simulink model "HVDCMMCInterconnection_O"  (R2023b)
settings: Solver=FixedStepDiscrete  StartTime=0.0  StopTime=10  RelTol=1e-3  EnableMultiTasking=on
PreLoadFcn:
  | HVDCMMCInterconnectionParam
StartFcn:
  | tic
StopFcn:
  | toc
values from neighbouring files (symbols this model uses):
  C_PM = 1.758e-3    (= 0.001758)    [HVDCMMCInterconnectionParam.m]
  Cfilter = 1/(Larm*wc2)    (= 4.78421193241e-05)    [HVDCMMCInterconnectionParam.m]
  Cg = 50e-9    (= 5e-08)    [HVDCMMCInterconnectionParam.m]
  Fc = Fnom*3.37    (= 168.5)    [HVDCMMCInterconnectionParam.m]
  Fnom = 50    [HVDCMMCInterconnectionParam.m]
  Ki_Ireg = 6    [HVDCMMCInterconnectionParam.m]
  Ki_Preg = 1.0    (= 1)    [HVDCMMCInterconnectionParam.m]
  Ki_Qreg = 1.0    (= 1)    [HVDCMMCInterconnectionParam.m]
  Ki_VDCreg = 100    [HVDCMMCInterconnectionParam.m]
  Kp_Ireg = 0.6    [HVDCMMCInterconnectionParam.m]
  Kp_Preg = 0.5/3    (= 0.166666666667)    [HVDCMMCInterconnectionParam.m]
  Kp_Qreg = 0.5/3    (= 0.166666666667)    [HVDCMMCInterconnectionParam.m]
  Kp_VDCreg = 4    [HVDCMMCInterconnectionParam.m]
  L_cable = 15e-3    (= 0.015)    [HVDCMMCInterconnectionParam.m]
  Larm = Larm_pu*(Zbase/(2*pi*Fnom))    (= 0.0529455974536)    [HVDCMMCInterconnectionParam.m]
  Lff = Larm_pu/2    (= 0.075)    [HVDCMMCInterconnectionParam.m]
  Limits_Ireg = [ 2.0  -2.0]    [HVDCMMCInterconnectionParam.m]
  Limits_Preg = [ 1.2, 0.8 ]    [HVDCMMCInterconnectionParam.m]
  Limits_Qreg = [ 0.25, -0.25 ]    [HVDCMMCInterconnectionParam.m]
  Limits_VDCreg = [ 2.0  -2.0]    [HVDCMMCInterconnectionParam.m]
  Lxfo = 0.12    [HVDCMMCInterconnectionParam.m]
  Nb_PM = 36    [HVDCMMCInterconnectionParam.m]
  Pnom = 1000e6    (= 1000000000)    [HVDCMMCInterconnectionParam.m]
  R_cable = 0.5    [HVDCMMCInterconnectionParam.m]
  R_startup = 400    [HVDCMMCInterconnectionParam.m]
  Rarm = Rarm_pu*Zbase    (= 0.1663335)    [HVDCMMCInterconnectionParam.m]
  Rff = Rarm_pu/2    (= 0.00075)    [HVDCMMCInterconnectionParam.m]
  Rfilter = 1/(Cfilter*w)*30    (= 1996.002)    [HVDCMMCInterconnectionParam.m]
  Rg = 100    [HVDCMMCInterconnectionParam.m]
  Rxfo = 0.003    [HVDCMMCInterconnectionParam.m]
  Slope_Pref = 0.5    [HVDCMMCInterconnectionParam.m]
  Slope_Qref = 0.5    [HVDCMMCInterconnectionParam.m]
  Slope_Vdc_ref = Vnom_dc/5    (= 128000)    [HVDCMMCInterconnectionParam.m]
  Tbrk1_On = 0.1    [HVDCMMCInterconnectionParam.m]
  Tbrk2_On = 1.0    (= 1)    [HVDCMMCInterconnectionParam.m]
  Tdeblock = 1.5    [HVDCMMCInterconnectionParam.m]
  Tfault = 9999    [HVDCMMCInterconnectionParam.m]
  Ton_Converter2 = 4    [HVDCMMCInterconnectionParam.m]
  Ton_PQreg = 4    [HVDCMMCInterconnectionParam.m]
  Ton_VDCreg = 1.5    [HVDCMMCInterconnectionParam.m]
  Ts = Ts_Control    (= 4e-05)    [HVDCMMCInterconnectionParam.m]
  Ts_Control = 40e-6    (= 4e-05)    [HVDCMMCInterconnectionParam.m]
  Ts_Power = 20e-6    (= 2e-05)    [HVDCMMCInterconnectionParam.m]
  Vnom_dc = 640e3    (= 640000)    [HVDCMMCInterconnectionParam.m]
  Vnom_prim = 400e3    (= 400000)    [HVDCMMCInterconnectionParam.m]
  Vnom_sec = 333e3    (= 333000)    [HVDCMMCInterconnectionParam.m]
undefined symbols (not defined in the file or in its folder): DiscIntNeverNeededParam, Pcc
libraries: spsSeriesRLCBranchLib x24, spsCurrentMeasurementLib x11, spsVoltageMeasurementLib x8, simulink x7, spsHalfBridgeMMCLib x6, powerlib_extras x3, spsIdealSwitchLib x3, spsBreakerLib x3, spsParallelRLCBranchLib x3, spsThreePhaseBreakerLib x2, spsMeanLib x2, spsSecondOrderFilterLib x2
(part 1 of 2)
settings Model: SimulationMode=accelerator  Creator=The MathWorks, Inc.  LastModifiedBy=The MathWorks, Inc.
settings SolverCC: AlgebraicLoopSolver=TrustRegion
settings DataIOCC: SaveFormat=StructureWithTime  SaveOutput=off  SignalLogging=off  DSMLogging=off  SaveTime=off  ReturnWorkspaceOutputs=off
settings OptimizationCC: ReuseModelBlockBuffer=off  ExpressionDepthLimit=2147483647  LifeSpan=inf
settings DebuggingCC: UnderspecifiedInitializationDetection=Classic  MergeDetectMultiDrivingBlocksExec=none  SolverPrmCheckMsg=warning  FcnCallInpInsideContextMsg=warning  UnconnectedInputMsg=warning  UnconnectedOutputMsg=warning  UnconnectedLineMsg=warning  AllowSymbolicDim=off  StateNameClashWarn=warning  SFUnexpectedBacktrackingDiag=warning  SFNoUnconditionalDefaultTransitionDiag=warning  SFExecutionAtInitializationDiag=none  ArithmeticOperatorsInVariantConditions=warning
settings HardwareCC: ProdBitPerPointer=32  ProdBitPerSizeT=32  ProdBitPerPtrDiffT=32  ProdLargestAtomicFloat=None  ProdIntDivRoundTo=Undefined  ProdEndianess=Unspecified  ProdWordSize=32  ProdHWDeviceType=32-bit Generic
settings ModelReferenceCC: EnableRefExpFcnMdlSchedulingChecks=on  PropagateSignalLabelsOutOfModel=off
settings SFSimCC: SimUseLocalCustomCode=off  CustomCodeUndefinedFunction=UseInterfaceOnly
settings RTWCC: RTWUseLocalCustomCode=off
settings CodeAppCC: StateflowObjectComments=on
settings GRTTargetCC: TargetLangStandard=C89/C90 (ANSI)  CombineOutputUpdateFcns=off  GRTInterface=on
settings ConfigComp: CovMetricSettings=dw  CovSaveCumulativeToWorkspaceVar=on  CovSaveSingleToWorkspaceVar=on  CovExternalEMLEnable=off
settings SimscapeCC: SimscapeNormalizeSystem=off

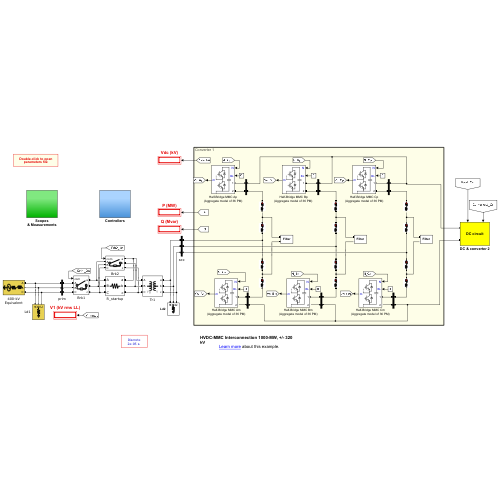
[thumbnail: Simulink's stored preview of the top-level diagram]
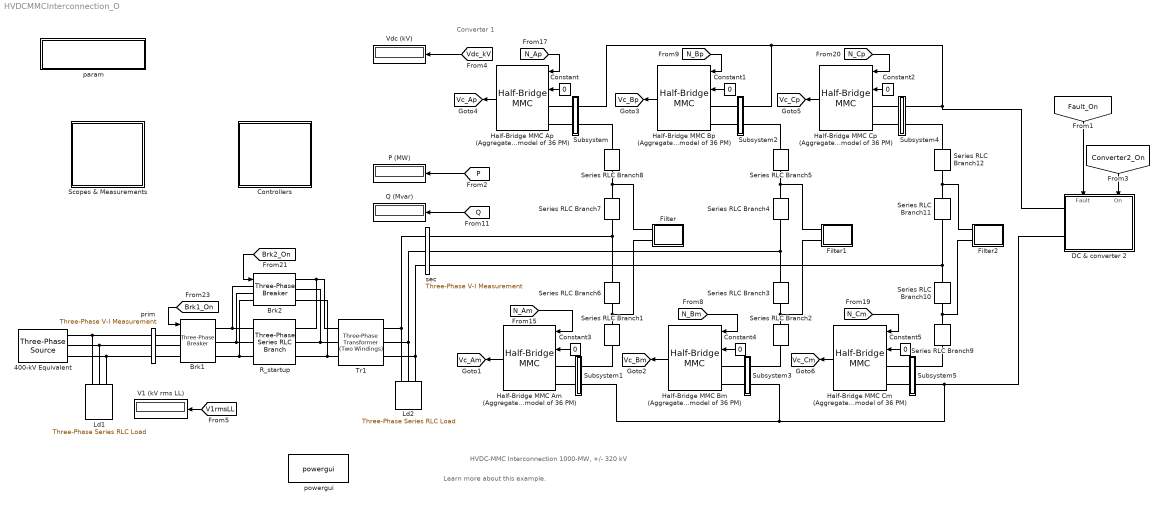
== system HVDCMMCInterconnection_O ==
  note: Converter 1
  note: HVDC-MMC Interconnection 1000-MW, +/- 320 kV
  note: Learn more about this example.
  400-kV Equivalent : spsThreePhaseSourceLib/Three-Phase Source  InternalConnection=Yg  VoltagePhases=off  Voltage=Vnom_prim*0.99  PhaseAngle=0  Voltage_phases=[25e3 25e3 25e3]/sqrt(3)  PhaseAngles_phases=[0 -120 +120]  Frequency=Fnom  NonIdealSource=on  SpecifyImpedance=on  Resistance=0.8929  Inductance=16.58e-3  ShortCircuitLevel=Psc  BaseVoltage=Vnom_prim  XRratio=7  BusType=swing  Pref=0  Qref=0  Prefabc=[10e3, 10e3, 10e3]  Qrefabc=[0, 0, 0]  Qmin=-inf  Qmax=inf
  Brk1 : spsThreePhaseBreakerLib/Three-Phase Breaker  InitialState=open  SwitchA=on  SwitchB=on  SwitchC=on  SwitchTimes=0.1  External=on  BreakerResistance=0.001  SnubberResistance=1e6  SnubberCapacitance=inf  Measurements=None
  Brk2 : spsThreePhaseBreakerLib/Three-Phase Breaker  InitialState=open  SwitchA=on  SwitchB=on  SwitchC=on  SwitchTimes=[30/60]*10000  External=on  BreakerResistance=0.01  SnubberResistance=1e6  SnubberCapacitance=inf  Measurements=None
  Constant{,1..5} (6 alike) : Constant  Value=0
  Controllers : Subsystem
  DC & converter 2 : Subsystem
      settings: PortSchema="{\"entries\":[{\"content\":{\"sides\":[{\"content\":{\"connectorIds\":[\"LConn1\",\"LConn2\"]},\"type\":\"ConnectorPlacement.EquallySpacedRectSide\",\"uuid\":\"7a2c87ad-91de-4512-ad2a-35713ffc2c67\"},{\"content\":{\"connectorIds\":[],\"side\":\"RIGHT\"},\"type\":\"ConnectorPlacement.EquallySpacedRectSide\",\"uuid\":\"a4d51b8d-9b80-4f56-8990-d227af10d4d9\"},{\"content\":{\"connectorIds\":[\"In1\",\"In2\"],\"side\":\"TOP\"},\"type\":\"ConnectorPlacement.EquallySpacedRectSide\",\"uuid\":\"21e823e1-439d-404c-83ef-6279f9df48a0\"}]},\"type\":\"ConnectorPlacement.EquallySpacedConnector\",\"uuid\":\"7be36849-7bc6-4892-aa95-a5e675f45e41\"}],\"packageUris\":[\"http://schema.mathworks.com/mf0/Connector/R2020b\"],\"version\":\"1.0\"}"
      mask Display: disp('DC circuit')
  Filter : Subsystem
      mask Display: disp('Filter')
  Filter1 : Subsystem
      mask Display: disp('Filter')
  Filter2 : Subsystem
      mask Display: disp('Filter')
  Half-Bridge MMC Am (Aggregate model of 36 PM) : spsHalfBridgeMMCLib/Half-Bridge MMC  ModelType=Aggregate model  n=36  C=C_PM  Vc_Initial=Vc0_PM  Ron=1e-3  Rs=1e6  Cs=inf  Ron_Diode=1e-3  Rs_Diode=1e6  Cs_Diode=inf  Vf_Diode=1e-3  Rs_CurrentSource=inf  Ts=Ts_Power
  Half-Bridge MMC Ap (Aggregate model of 36 PM) : spsHalfBridgeMMCLib/Half-Bridge MMC  ModelType=Aggregate model  n=36  C=C_PM  Vc_Initial=Vc0_PM  Ron=1e-3  Rs=1e6  Cs=inf  Ron_Diode=1e-3  Rs_Diode=1e6  Cs_Diode=inf  Vf_Diode=1e-3  Rs_CurrentSource=inf  Ts=Ts_Power
  Half-Bridge MMC Bm (Aggregate model of 36 PM) : spsHalfBridgeMMCLib/Half-Bridge MMC  ModelType=Aggregate model  n=36  C=C_PM  Vc_Initial=Vc0_PM  Ron=1e-3  Rs=1e6  Cs=inf  Ron_Diode=1e-3  Rs_Diode=1e6  Cs_Diode=inf  Vf_Diode=1e-3  Rs_CurrentSource=inf  Ts=Ts_Power
  "Half-Bridge MMC Bp (Aggregate model of 36 PM) " : spsHalfBridgeMMCLib/Half-Bridge MMC  ModelType=Aggregate model  n=36  C=C_PM  Vc_Initial=Vc0_PM  Ron=1e-3  Rs=1e6  Cs=inf  Ron_Diode=1e-3  Rs_Diode=1e6  Cs_Diode=inf  Vf_Diode=1e-3  Rs_CurrentSource=inf  Ts=Ts_Power
  Half-Bridge MMC Cm (Aggregate model of 36 PM) : spsHalfBridgeMMCLib/Half-Bridge MMC  ModelType=Aggregate model  n=36  C=C_PM  Vc_Initial=Vc0_PM  Ron=1e-3  Rs=1e6  Cs=inf  Ron_Diode=1e-3  Rs_Diode=1e6  Cs_Diode=inf  Vf_Diode=1e-3  Rs_CurrentSource=inf  Ts=Ts_Power
  Half-Bridge MMC Cp (Aggregate model of 36 PM) : spsHalfBridgeMMCLib/Half-Bridge MMC  ModelType=Aggregate model  n=36  C=C_PM  Vc_Initial=Vc0_PM  Ron=1e-3  Rs=1e6  Cs=inf  Ron_Diode=1e-3  Rs_Diode=1e6  Cs_Diode=inf  Vf_Diode=1e-3  Rs_CurrentSource=inf  Ts=Ts_Power
  Ld1 : spsThreePhaseSeriesRLCLoadLib/Three-Phase Series RLC Load  LConnTagsString=A|B|C  Configuration=Y (grounded)  NominalVoltage=Vnom_prim  Vabc=[1e3 1e3 1e3]  Vabcp=[1e3 1e3 1e3]  NominalFrequency=Fnom  UnbalancedPower=off  ActivePower=P_Ld1  InductivePower=0  CapacitivePower=0  Pabc=[10e3 9e3 11e3]  QLabc=[100 90 110]  QCabc=[100 90 110]  Pabcp=[10e3 9e3 11e3]  QLabcp=[100 90 110]  QCabcp=[100 90 110]  Measurements=None  LoadType=constant Z
  Ld2 : spsThreePhaseSeriesRLCLoadLib/Three-Phase Series RLC Load  LConnTagsString=A|B|C  Configuration=Y (grounded)  NominalVoltage=Vnom_sec  Vabc=[1e3 1e3 1e3]  Vabcp=[1e3 1e3 1e3]  NominalFrequency=Fnom  UnbalancedPower=off  ActivePower=500e3  InductivePower=0  CapacitivePower=0  Pabc=[10e3 9e3 11e3]  QLabc=[100 90 110]  QCabc=[100 90 110]  Pabcp=[10e3 9e3 11e3]  QLabcp=[100 90 110]  QCabcp=[100 90 110]  Measurements=None  LoadType=constant Z
  P (MW) : Display
      settings: Format=bank  Decimation=5000
  Q (Mvar) : Display
      settings: Format=bank  Decimation=5000
  R_startup : spsThreePhaseSeriesRLCBranchLib/Three-Phase Series RLC Branch  LConnTagsString=A|B|C  RConnTagsString=A|B|C  BranchType=R  Resistance=R_startup  Inductance=Vnom_prim^2 / Pcc / (2*pi*Fnom)  Capacitance=1e-6  Measurements=None
  Scopes & Measurements : Subsystem
  Series RLC Branch{1..12} (12 alike) : spsSeriesRLCBranchLib/Series RLC Branch  LConnTagsString=__new0  RConnTagsString=__new0  BranchType=RL  Resistance=Rarm/2  Inductance=Larm/2  SetiL0=off  InitialCurrent=0  Capacitance=1e-6  Setx0=off  InitialVoltage=0  Measurements=None
  Subsystem : Subsystem
  Subsystem1 : Subsystem
  Subsystem2 : Subsystem
  Subsystem3 : Subsystem
  Subsystem4 : Subsystem
  Subsystem5 : Subsystem
  Tr1 : spsThreePhaseTransformerTwoWindingsLib/Three-Phase Transformer (Two Windings)  Winding1Connection=Yg  Winding2Connection=Y  CoreType=Three single-phase transformers  SetSaturation=off  Hysteresis=off  DataFile='hysteresis'  SetInitialFlux=off  Measurements=None  UNITS=pu  NominalPower=[ Pnom , Fnom ]  Winding1="[ Vnom_prim , Rxfo/2,  Lxfo/2 ]"  Winding2="[ Vnom_sec , Rxfo/2,  Lxfo/2 ]"  Rm=1000  Lm=1000  L0=0.5  Saturation=[ 0,0 ; 0.0024,1.2 ; 1.0,1.52 ]  InitialFluxes=[ 0.8 , -0.8 , 0.7 ]  BreakLoop=off  DiscreteSolver=Trapezoidal iterative  DataType=off  TransfoNumber=1
  V1 (kV rms LL) : Display
      settings: Format=bank  Decimation=5000
  Vdc (kV) : Display
      settings: Format=bank  Decimation=5000
  param : Subsystem
      settings: OpenFcn=open('HVDCMMCInterconnectionParam')
      mask Display: disp('Double-click to open\nparameters file')
  powergui : spspowerguiLib/powergui  Priority=1  SimulationMode=Discrete  SampleTime=Ts_Power  frequency=60  Iterations=50  frequencyindice=0  Pbase=100e6  ErrMax=1e-4  UnitsV=kV  UnitsW=MW  buscounter=0  FunctionMessages=off  echomessages=off  EnableUseOfTLC=off  CurrentSourceSwitches=off  DisableSnubberDevices=off  DisableRonSwitches=off  DisableVfSwitches=off  DisplayEquations=off  AutomaticDiscreteSolvers=off  SolverType=Tustin/Backward Euler (TBE)  Interpol=off  ExternalGateDelay=off  methode=off  Ts=10  x0status=blocks  SPID=off  SwTol=0  HookPort=off  NonlinearTolerance=1e-4  nMaxIteration=100  ContinueOnMaxIteration=off  RestoreLinks=warning  ResistiveCurrentMeasurement=off  Frange=[0:2:500]  Ylog=off  Xlog=on  ShowGrid=off  save=off  variable=ZData  structure=VIprim  ZoomFFT=on  StartTime=0.15  cycles=2  DisplayStyle=1  fundamental=50  FreqAxis=on  MaxFrequency=1000  frequencyindicesteady=1  RmsSteady=1  display=off
  prim : spsThreePhaseVIMeasurementLib/Three-Phase V-I Measurement  VoltageMeasurement=phase-to-ground  SetLabelV=on  LabelV=Vprim  Vpu=off  VpuLL=off  CurrentMeasurement=yes  SetLabelI=on  LabelI=Iprim  Ipu=off  Pbase=100e6  Vbase=500e3  OutputType=Complex  PhasorSimulation=off  PSBequivalent=0
  sec : spsThreePhaseVIMeasurementLib/Three-Phase V-I Measurement  VoltageMeasurement=phase-to-ground  SetLabelV=on  LabelV=Vsec  Vpu=off  VpuLL=off  CurrentMeasurement=yes  SetLabelI=on  LabelI=Isec  Ipu=off  Pbase=100e6  Vbase=500e3  OutputType=Complex  PhasorSimulation=off  PSBequivalent=0
  tag scope: Vc_Am=global, Vc_Ap=global, Vc_Bm=global, Vc_Bp=global, Vc_Cm=global, Vc_Cp=global
  wires:
  [P] -> P (MW)/1
  [N_Cp] -> Half-Bridge MMC Cp (Aggregate model of 36 PM)/1
  Half-Bridge MMC Cp (Aggregate model of 36 PM)/1 -> [Vc_Cp]
  Half-Bridge MMC Am (Aggregate model of 36 PM)/1 -> [Vc_Am]
  Half-Bridge MMC Bm (Aggregate model of 36 PM)/1 -> [Vc_Bm]
  Half-Bridge MMC Cm (Aggregate model of 36 PM)/1 -> [Vc_Cm]
  [N_Bm] -> Half-Bridge MMC Bm (Aggregate model of 36 PM)/1
  [Brk2_On] -> Brk2/1
  [Brk1_On] -> Brk1/1
  [Vdc_kV] -> Vdc (kV)/1
  [V1rmsLL] -> V1 (kV rms LL)/1
  [Q] -> Q (Mvar)/1
  Half-Bridge MMC Ap (Aggregate model of 36 PM)/1 -> [Vc_Ap]
  [Converter2_On] -> DC & converter 2/2(On)
  [Fault_On] -> DC & converter 2/1(Fault)
  [N_Ap] -> Half-Bridge MMC Ap (Aggregate model of 36 PM)/1
  [N_Am] -> Half-Bridge MMC Am (Aggregate model of 36 PM)/1
  "Half-Bridge MMC Bp (Aggregate model of 36 PM) "/1 -> [Vc_Bp]
  [N_Bp] -> "Half-Bridge MMC Bp (Aggregate model of 36 PM) "/1
  [N_Cm] -> Half-Bridge MMC Cm (Aggregate model of 36 PM)/1
  Constant/1 -> Half-Bridge MMC Ap (Aggregate model of 36 PM)/2
  Constant1/1 -> "Half-Bridge MMC Bp (Aggregate model of 36 PM) "/2
  Constant2/1 -> Half-Bridge MMC Cp (Aggregate model of 36 PM)/2
  Constant3/1 -> Half-Bridge MMC Am (Aggregate model of 36 PM)/2
  Constant4/1 -> Half-Bridge MMC Bm (Aggregate model of 36 PM)/2
  Constant5/1 -> Half-Bridge MMC Cm (Aggregate model of 36 PM)/2
  connections:
  400-kV Equivalent/RConn1 -- Ld1/LConn1 -- prim/RConn1
  400-kV Equivalent/RConn2 -- Ld1/LConn2 -- prim/RConn2
  400-kV Equivalent/RConn3 -- Ld1/LConn3 -- prim/RConn3
  Series RLC Branch7/RConn1 -- Series RLC Branch6/LConn1 -- sec/LConn1
  Series RLC Branch1/LConn1 -- Filter/LConn2 -- Series RLC Branch6/RConn1
  Series RLC Branch7/LConn1 -- Filter/LConn1 -- Series RLC Branch8/RConn1
  Half-Bridge MMC Ap (Aggregate model of 36 PM)/LConn1 -- Subsystem/LConn1
  Subsystem/LConn2 -- Half-Bridge MMC Ap (Aggregate model of 36 PM)/LConn2
  Subsystem/RConn2 -- Series RLC Branch8/LConn1
  Half-Bridge MMC Am (Aggregate model of 36 PM)/LConn2 -- Subsystem1/LConn2
  Half-Bridge MMC Am (Aggregate model of 36 PM)/LConn1 -- Subsystem1/LConn1
  Series RLC Branch1/RConn1 -- Subsystem1/RConn1
  Series RLC Branch4/RConn1 -- Series RLC Branch3/LConn1 -- sec/LConn2
  Filter1/LConn2 -- Series RLC Branch2/LConn1 -- Series RLC Branch3/RConn1
  Series RLC Branch4/LConn1 -- Filter1/LConn1 -- Series RLC Branch5/RConn1
  "Half-Bridge MMC Bp (Aggregate model of 36 PM) "/LConn2 -- Subsystem2/LConn2
  "Half-Bridge MMC Bp (Aggregate model of 36 PM) "/LConn1 -- Subsystem2/LConn1
  Subsystem2/RConn2 -- Series RLC Branch5/LConn1
  Series RLC Branch2/RConn1 -- Subsystem3/RConn1
  Half-Bridge MMC Bm (Aggregate model of 36 PM)/LConn1 -- Subsystem3/LConn1
  Half-Bridge MMC Bm (Aggregate model of 36 PM)/LConn2 -- Subsystem3/LConn2
  Series RLC Branch11/RConn1 -- Series RLC Branch10/LConn1 -- sec/LConn3
  Series RLC Branch10/RConn1 -- Filter2/LConn2 -- Series RLC Branch9/LConn1
  Series RLC Branch12/RConn1 -- Series RLC Branch11/LConn1 -- Filter2/LConn1
  Half-Bridge MMC Cp (Aggregate model of 36 PM)/LConn1 -- Subsystem4/LConn1
  Half-Bridge MMC Cm (Aggregate model of 36 PM)/LConn1 -- Subsystem5/LConn1
  Half-Bridge MMC Cm (Aggregate model of 36 PM)/LConn2 -- Subsystem5/LConn2
  Subsystem4/RConn2 -- Series RLC Branch12/LConn1
  Half-Bridge MMC Cp (Aggregate model of 36 PM)/LConn2 -- Subsystem4/LConn2
  Series RLC Branch9/RConn1 -- Subsystem5/RConn1
  Subsystem/RConn1 -- Subsystem4/RConn1 -- DC & converter 2/LConn1 -- Subsystem2/RConn1
  Subsystem1/RConn2 -- Subsystem5/RConn2 -- DC & converter 2/LConn2 -- Subsystem3/RConn2
  sec/RConn1 -- Ld2/LConn1 -- Tr1/RConn1
  sec/RConn2 -- Ld2/LConn2 -- Tr1/RConn2
  sec/RConn3 -- Ld2/LConn3 -- Tr1/RConn3
  Brk2/LConn1 -- R_startup/LConn1 -- Brk1/RConn1
  Brk1/RConn2 -- Brk2/LConn2 -- R_startup/LConn2
  Brk1/RConn3 -- Brk2/LConn3 -- R_startup/LConn3
  R_startup/RConn1 -- Brk2/RConn1 -- Tr1/LConn1
  R_startup/RConn2 -- Brk2/RConn2 -- Tr1/LConn2
  R_startup/RConn3 -- Brk2/RConn3 -- Tr1/LConn3
  prim/LConn1 -- Brk1/LConn1
  prim/LConn2 -- Brk1/LConn2
  prim/LConn3 -- Brk1/LConn3

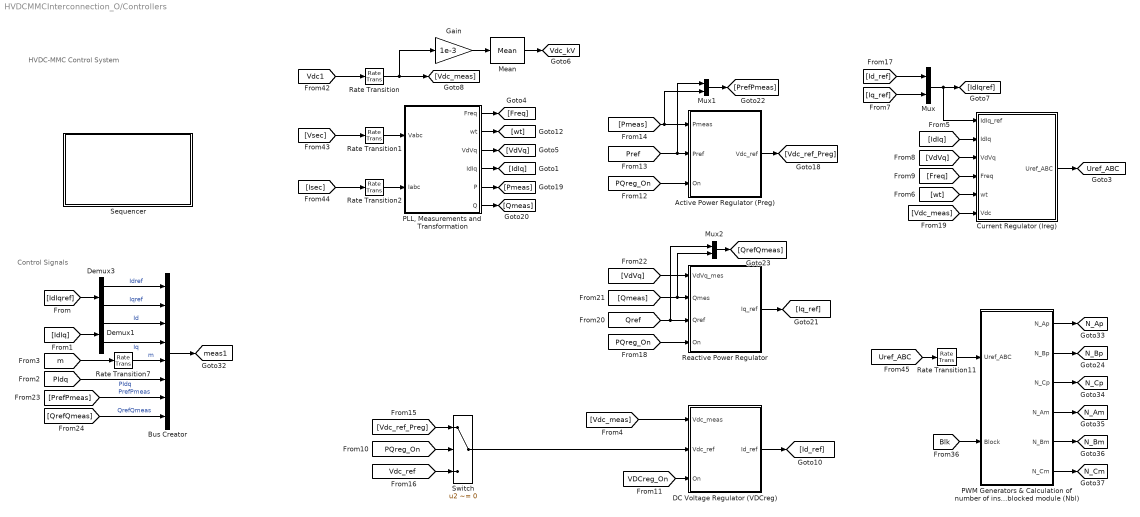
== system HVDCMMCInterconnection_O/Controllers ==
  note: HVDC-MMC Control System
  note: Control Signals
  Active Power Regulator (Preg) : Subsystem
  Bus Creator : BusCreator  Inputs=8
  Current Regulator (Ireg) : Subsystem
  DC Voltage Regulator (VDCreg) : Subsystem
  Demux1 : Demux  Outputs=2
  Demux3 : Demux  Outputs=2
  Gain : Gain  Gain=1e-3
  Mean : spsMeanLib/Mean  Freq=Fnom/3  Vinit=0  Ts=Ts_Control
  Mux : Mux  Inputs=2
  Mux1 : Mux  Inputs=2
  Mux2 : Mux  Inputs=2
  "PLL, Measurements and Transformation" : Subsystem
  PWM Generators & Calculation of number of inserted modules (Nin) and number of blocked module (Nbl) : Subsystem
  Rate Transition{,1..2,7} (4 alike) : RateTransition  OutPortSampleTime=Ts_Control
  Rate Transition11 : RateTransition  OutPortSampleTime=Ts_Power
  Reactive Power Regulator : Subsystem
  Sequencer : Subsystem
      mask Display: disp('Sequencer')
  Switch : Switch  Criteria=u2 ~= 0  SaturateOnIntegerOverflow=off  InputSameDT=off
  tag scope: N_Am=global, N_Ap=global, N_Bm=global, N_Bp=global, N_Cm=global, N_Cp=global, Uref_ABC=global, Vdc_kV=global, meas1=global
  wires:
  Rate Transition11/1 -> PWM Generators & Calculation of number of inserted modules (Nin) and number of blocked module (Nbl)/1(Uref_ABC)
  [Uref_ABC] -> Rate Transition11/1
  Mean/1 -> [Vdc_kV]
  [Vsec] -> Rate Transition1/1
  [Isec] -> Rate Transition2/1
  [Vdc_meas] -> Current Regulator (Ireg)/6(Vdc)
  [Vdc_meas] -> DC Voltage Regulator (VDCreg)/1(Vdc_meas)
  DC Voltage Regulator (VDCreg)/1(Id_ref) -> [Id_ref]
  Gain/1 -> Mean/1
  Current Regulator (Ireg)/1(Uref_ABC) -> [Uref_ABC]
  [wt] -> Current Regulator (Ireg)/5(wt)
  [Vdc1] -> Rate Transition/1
  "PLL, Measurements and Transformation"/2(wt) -> [wt]
  "PLL, Measurements and Transformation"/4(IdIq) -> [IdIq]
  [Freq] -> Current Regulator (Ireg)/4(Freq)
  [Id_ref] -> Mux/1
  "PLL, Measurements and Transformation"/3(VdVq) -> [VdVq]
  Mux/1 -> Current Regulator (Ireg)/1(IdIq_ref), [IdIqref]
  Demux1/2 -> Bus Creator/4  "Iq"
  [IdIq] -> Current Regulator (Ireg)/2(IdIq)
  [IdIqref] -> Demux3/1
  Demux3/1 -> Bus Creator/1  "Idref"
  [IdIq] -> Demux1/1
  Bus Creator/1 -> [meas1]
  Demux3/2 -> Bus Creator/2  "Iqref"
  [m] -> Rate Transition7/1
  Demux1/1 -> Bus Creator/3  "Id"
  [PIdq] -> Bus Creator/6  "PIdq"
  "PLL, Measurements and Transformation"/1(Freq) -> [Freq]
  [VdVq] -> Current Regulator (Ireg)/3(VdVq)
  [Iq_ref] -> Mux/2
  Rate Transition/1 -> Gain/1, [Vdc_meas]
  Rate Transition2/1 -> "PLL, Measurements and Transformation"/2(Iabc)
  Rate Transition7/1 -> Bus Creator/5  "m"
  Rate Transition1/1 -> "PLL, Measurements and Transformation"/1(Vabc)
  [Vdc_ref] -> Switch/3
  [PQreg_On] -> Reactive Power Regulator/4(On)
  Mux2/1 -> [QrefQmeas]
  Mux1/1 -> [PrefPmeas]
  [Vdc_ref_Preg] -> Switch/1
  [Qref] -> Mux2/1, Reactive Power Regulator/3(Qref)
  [QrefQmeas] -> Bus Creator/8  "QrefQmeas"
  [VDCreg_On] -> DC Voltage Regulator (VDCreg)/3(On)
  [PQreg_On] -> Active Power Regulator (Preg)/3(On)
  Active Power Regulator (Preg)/1(Vdc_ref) -> [Vdc_ref_Preg]
  Reactive Power Regulator/1(Iq_ref) -> [Iq_ref]
  "PLL, Measurements and Transformation"/5(P) -> [Pmeas]
  [VdVq] -> Reactive Power Regulator/1(VdVq_mes)
  [Qmeas] -> Mux2/2, Reactive Power Regulator/2(Qmes)
  [PQreg_On] -> Switch/2
  Switch/1 -> DC Voltage Regulator (VDCreg)/2(Vdc_ref)
  [Pref] -> Active Power Regulator (Preg)/2(Pref), Mux1/1
  [PrefPmeas] -> Bus Creator/7  "PrefPmeas"
  "PLL, Measurements and Transformation"/6(Q) -> [Qmeas]
  [Pmeas] -> Active Power Regulator (Preg)/1(Pmeas), Mux1/2
  PWM Generators & Calculation of number of inserted modules (Nin) and number of blocked module (Nbl)/1(N_Ap) -> [N_Ap]
  PWM Generators & Calculation of number of inserted modules (Nin) and number of blocked module (Nbl)/2(N_Bp) -> [N_Bp]
  PWM Generators & Calculation of number of inserted modules (Nin) and number of blocked module (Nbl)/3(N_Cp) -> [N_Cp]
  PWM Generators & Calculation of number of inserted modules (Nin) and number of blocked module (Nbl)/4(N_Am) -> [N_Am]
  PWM Generators & Calculation of number of inserted modules (Nin) and number of blocked module (Nbl)/5(N_Bm) -> [N_Bm]
  PWM Generators & Calculation of number of inserted modules (Nin) and number of blocked module (Nbl)/6(N_Cm) -> [N_Cm]
  [Blk] -> PWM Generators & Calculation of number of inserted modules (Nin) and number of blocked module (Nbl)/2(Block)

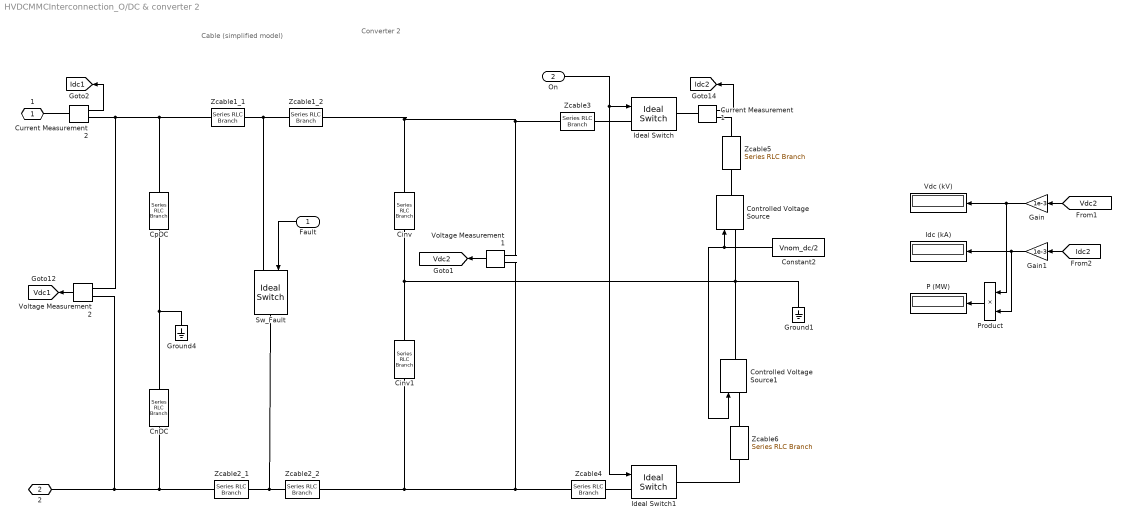
== system HVDCMMCInterconnection_O/DC & converter 2 ==
  note: Cable (simplified model)
  note: Converter 2
  Fault : Inport
  On : Inport  Port=2
  Cinv : spsSeriesRLCBranchLib/Series RLC Branch  LConnTagsString=__new0  RConnTagsString=__new0  BranchType=RC  Resistance=1e-3  Inductance=1e-3  SetiL0=off  InitialCurrent=0  Capacitance=C_PM/Nb_PM*3  Setx0=off  InitialVoltage=Vnom_dc/2  Measurements=None
  Cinv1 : spsSeriesRLCBranchLib/Series RLC Branch  LConnTagsString=__new0  RConnTagsString=__new0  BranchType=RC  Resistance=1e-3  Inductance=1e-3  SetiL0=off  InitialCurrent=0  Capacitance=C_PM/Nb_PM*3  Setx0=off  InitialVoltage=Vnom_dc/2  Measurements=None
  CnDC : spsSeriesRLCBranchLib/Series RLC Branch  LConnTagsString=__new0  RConnTagsString=__new0  BranchType=RC  Resistance=Rg  Inductance=1e-3  SetiL0=off  InitialCurrent=0  Capacitance=Cg  Setx0=off  InitialVoltage=Vnom_dc/2  Measurements=None
  Constant2 : Constant  Value=Vnom_dc/2  SampleTime=Ts_Power
  Controlled Voltage Source : spsControlledVoltageSourceLib/Controlled Voltage Source  Initialize=off  Source_Type=AC  Amplitude=0  Phase=0  Frequency=0  Measurements=None
  Controlled Voltage Source1 : spsControlledVoltageSourceLib/Controlled Voltage Source  Initialize=off  Source_Type=AC  Amplitude=0  Phase=0  Frequency=0  Measurements=None
  CpDC : spsSeriesRLCBranchLib/Series RLC Branch  LConnTagsString=__new0  RConnTagsString=__new0  BranchType=RC  Resistance=Rg  Inductance=1e-3  SetiL0=off  InitialCurrent=0  Capacitance=Cg  Setx0=off  InitialVoltage=Vnom_dc/2  Measurements=None
  Current Measurement1 : spsCurrentMeasurementLib/Current Measurement  PhasorSimulation=off  OutputType=Complex  PSBequivalent=0
  Current Measurement2 : spsCurrentMeasurementLib/Current Measurement  PhasorSimulation=off  OutputType=Complex  PSBequivalent=0
  Gain : Gain  Gain=1e-3
  Gain1 : Gain  Gain=1e-3
  Ground1 : spsGroundLib/Ground  LConnTagsString=a
  Ground4 : spsGroundLib/Ground  LConnTagsString=a
  Idc (kA) : Display
      settings: Format=bank  Decimation=5000
  Ideal Switch : spsIdealSwitchLib/Ideal Switch  Ron=0.001  Lon=0  IC=0  Rs=1e6  Cs=inf  Measurements=off
  Ideal Switch1 : spsIdealSwitchLib/Ideal Switch  Ron=0.001  Lon=0  IC=0  Rs=1e6  Cs=inf  Measurements=off
  P (MW) : Display
      settings: Format=bank  Decimation=5000
  Product : Product
  Sw_Fault : spsIdealSwitchLib/Ideal Switch  Ron=Rfault  Lon=0  IC=0  Rs=1e6  Cs=inf  Measurements=off
  Vdc (kV) : Display
      settings: Format=bank  Decimation=5000
  Voltage Measurement1 : spsVoltageMeasurementLib/Voltage Measurement  PhasorSimulation=off  OutputType=Complex  PSBequivalent=0
  Voltage Measurement2 : spsVoltageMeasurementLib/Voltage Measurement  PhasorSimulation=off  OutputType=Complex  PSBequivalent=0
  Zcable1_1 : spsSeriesRLCBranchLib/Series RLC Branch  LConnTagsString=__new0  RConnTagsString=__new0  BranchType=RL  Resistance=R_cable/2  Inductance=L_cable/2  SetiL0=off  InitialCurrent=0  Capacitance=1e-6  Setx0=off  InitialVoltage=0  Measurements=None
  Zcable1_2 : spsSeriesRLCBranchLib/Series RLC Branch  LConnTagsString=__new0  RConnTagsString=__new0  BranchType=RL  Resistance=R_cable/2  Inductance=L_cable/2  SetiL0=off  InitialCurrent=0  Capacitance=1e-6  Setx0=off  InitialVoltage=0  Measurements=None
  Zcable2_1 : spsSeriesRLCBranchLib/Series RLC Branch  LConnTagsString=__new0  RConnTagsString=__new0  BranchType=RL  Resistance=R_cable/2  Inductance=L_cable/2  SetiL0=off  InitialCurrent=0  Capacitance=1e-6  Setx0=off  InitialVoltage=0  Measurements=None
  Zcable2_2 : spsSeriesRLCBranchLib/Series RLC Branch  LConnTagsString=__new0  RConnTagsString=__new0  BranchType=RL  Resistance=R_cable/2  Inductance=L_cable/2  SetiL0=off  InitialCurrent=0  Capacitance=1e-6  Setx0=off  InitialVoltage=0  Measurements=None
  Zcable3 : spsSeriesRLCBranchLib/Series RLC Branch  LConnTagsString=__new0  RConnTagsString=__new0  BranchType=R  Resistance=1e-3  Inductance=1e-3  SetiL0=off  InitialCurrent=0  Capacitance=1e-6  Setx0=off  InitialVoltage=0  Measurements=None
  Zcable4 : spsSeriesRLCBranchLib/Series RLC Branch  LConnTagsString=__new0  RConnTagsString=__new0  BranchType=R  Resistance=1e-3  Inductance=1e-3  SetiL0=off  InitialCurrent=0  Capacitance=1e-6  Setx0=off  InitialVoltage=0  Measurements=None
  Zcable5 : spsSeriesRLCBranchLib/Series RLC Branch  LConnTagsString=__new0  RConnTagsString=__new0  BranchType=RL  Resistance=1e-2  Inductance=1e-4  SetiL0=off  InitialCurrent=0  Capacitance=1e-6  Setx0=off  InitialVoltage=0  Measurements=None
  Zcable6 : spsSeriesRLCBranchLib/Series RLC Branch  LConnTagsString=__new0  RConnTagsString=__new0  BranchType=RL  Resistance=1e-2  Inductance=1e-4  SetiL0=off  InitialCurrent=0  Capacitance=1e-6  Setx0=off  InitialVoltage=0  Measurements=None
  1 : PMIOPort  Side=Left
  2 : PMIOPort  Port=2  Side=Left
  tag scope: Idc1=global, Idc2=global, Vdc1=global, Vdc2=global
  wires:
  Voltage Measurement2/1 -> [Vdc1]
  Constant2/1 -> Controlled Voltage Source1/1, Controlled Voltage Source/1
  Voltage Measurement1/1 -> [Vdc2]
  Gain/1 -> Product/1, Vdc (kV)/1
  Gain1/1 -> Product/2, Idc (kA)/1
  [Vdc2] -> Gain/1
  [Idc2] -> Gain1/1
  Product/1 -> P (MW)/1
  Current Measurement1/1 -> [Idc2]
  Current Measurement2/1 -> [Idc1]
  On/1 -> Ideal Switch1/1, Ideal Switch/1
  Fault/1 -> Sw_Fault/1
  connections:
  Voltage Measurement1/LConn1 -- Zcable1_2/LConn1 -- Cinv/LConn1 -- Zcable3/RConn1
  Controlled Voltage Source1/RConn1 -- Ground1/LConn1 -- Cinv1/LConn1 -- Cinv/RConn1 -- Controlled Voltage Source/LConn1
  Ground4/LConn1 -- CnDC/LConn1 -- CpDC/RConn1
  Zcable2_1/RConn1 -- CnDC/RConn1 -- Voltage Measurement2/LConn2 -- 2/RConn1
  Zcable2_2/RConn1 -- Sw_Fault/RConn1 -- Zcable2_1/LConn1
  Ideal Switch/LConn1 -- Zcable3/LConn1
  Ideal Switch1/LConn1 -- Zcable4/LConn1
  Zcable1_1/RConn1 -- Voltage Measurement2/LConn1 -- Current Measurement2/RConn1 -- CpDC/LConn1
  Ideal Switch/RConn1 -- Current Measurement1/LConn1
  Zcable5/LConn1 -- Current Measurement1/RConn1
  Zcable5/RConn1 -- Controlled Voltage Source/RConn1
  Zcable6/LConn1 -- Controlled Voltage Source1/LConn1
  Zcable6/RConn1 -- Ideal Switch1/RConn1
  1/RConn1 -- Current Measurement2/LConn1
  Zcable1_1/LConn1 -- Zcable1_2/RConn1 -- Sw_Fault/LConn1
  Zcable2_2/LConn1 -- Cinv1/RConn1 -- Zcable4/RConn1 -- Voltage Measurement1/LConn2

== system HVDCMMCInterconnection_O/Filter ==
  Breaker : spsBreakerLib/Breaker  InitialState=1  SwitchingTimes=Topen_Filter  External=off  BreakerResistance=0.001  SnubberResistance=1e6  SnubberCapacitance=inf  Measurements=None  MoreParameters=on  NoBreakLoop=off
  Current Measurement6 : spsCurrentMeasurementLib/Current Measurement  PhasorSimulation=off  OutputType=Complex  PSBequivalent=0
  Parallel RLC Branch : spsParallelRLCBranchLib/Parallel RLC Branch  LConnTagsString=a  RConnTagsString=__new0  BranchType=RC  Resistance=Rfilter  Inductance=1e-3  SetiL0=off  InitialCurrent=0  Capacitance=Cfilter  Setx0=off  InitialVoltage=0  Measurements=None
  1 : PMIOPort  Side=Left
  2 : PMIOPort  Port=2  Side=Left
  tag scope: Ifilter_A=global
  wires:
  Current Measurement6/1 -> [Ifilter_A]
  connections:
  Parallel RLC Branch/RConn1 -- 2/RConn1
  Current Measurement6/RConn1 -- Parallel RLC Branch/LConn1
  1/RConn1 -- Breaker/LConn1
  Breaker/RConn1 -- Current Measurement6/LConn1

== system HVDCMMCInterconnection_O/Filter1 ==
  Breaker : spsBreakerLib/Breaker  InitialState=1  SwitchingTimes=Topen_Filter  External=off  BreakerResistance=0.001  SnubberResistance=1e6  SnubberCapacitance=inf  Measurements=None  MoreParameters=on  NoBreakLoop=off
  Current Measurement6 : spsCurrentMeasurementLib/Current Measurement  PhasorSimulation=off  OutputType=Complex  PSBequivalent=0
  Parallel RLC Branch : spsParallelRLCBranchLib/Parallel RLC Branch  LConnTagsString=a  RConnTagsString=__new0  BranchType=RC  Resistance=Rfilter  Inductance=1e-3  SetiL0=off  InitialCurrent=0  Capacitance=Cfilter  Setx0=off  InitialVoltage=0  Measurements=None
  1 : PMIOPort  Side=Left
  2 : PMIOPort  Port=2  Side=Left
  tag scope: Ifilter_B=global
  wires:
  Current Measurement6/1 -> [Ifilter_B]
  connections:
  Current Measurement6/RConn1 -- Parallel RLC Branch/LConn1
  Parallel RLC Branch/RConn1 -- 2/RConn1
  1/RConn1 -- Breaker/LConn1
  Breaker/RConn1 -- Current Measurement6/LConn1

== system HVDCMMCInterconnection_O/Filter2 ==
  Breaker : spsBreakerLib/Breaker  InitialState=1  SwitchingTimes=Topen_Filter  External=off  BreakerResistance=0.001  SnubberResistance=1e6  SnubberCapacitance=inf  Measurements=None  MoreParameters=on  NoBreakLoop=off
  Current Measurement6 : spsCurrentMeasurementLib/Current Measurement  PhasorSimulation=off  OutputType=Complex  PSBequivalent=0
  Parallel RLC Branch : spsParallelRLCBranchLib/Parallel RLC Branch  LConnTagsString=a  RConnTagsString=__new0  BranchType=RC  Resistance=Rfilter  Inductance=1e-3  SetiL0=off  InitialCurrent=0  Capacitance=Cfilter  Setx0=off  InitialVoltage=0  Measurements=None
  1 : PMIOPort  Side=Left
  2 : PMIOPort  Port=2  Side=Left
  tag scope: Ifilter_C=global
  wires:
  Current Measurement6/1 -> [Ifilter_C]
  connections:
  Parallel RLC Branch/RConn1 -- 2/RConn1
  Current Measurement6/RConn1 -- Parallel RLC Branch/LConn1
  Current Measurement6/LConn1 -- Breaker/RConn1
  1/RConn1 -- Breaker/LConn1

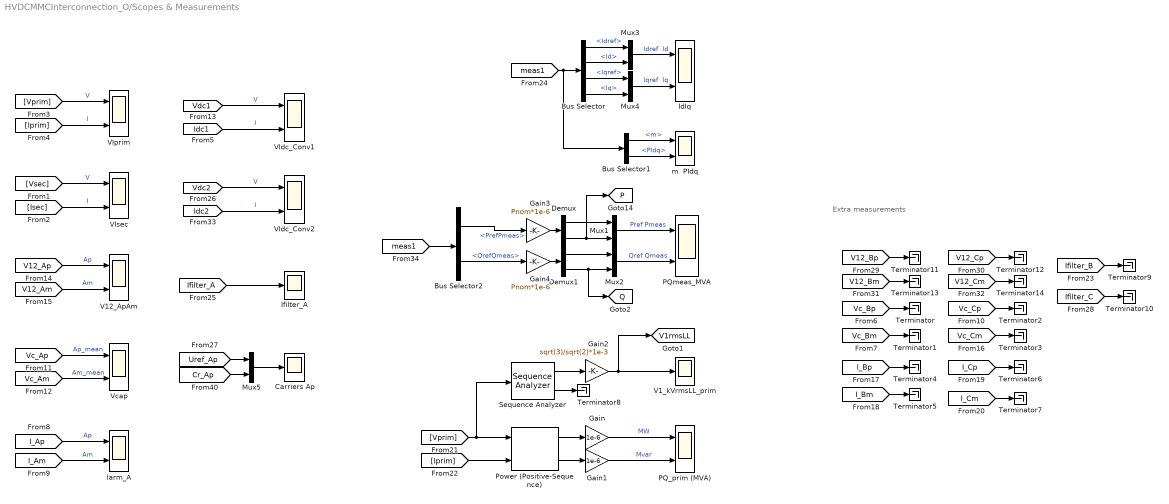
== system HVDCMMCInterconnection_O/Scopes & Measurements ==
  note: Extra measurements
  Bus Selector : BusSelector  OutputSignals=Idref,Id,Iqref,Iq
  Bus Selector1 : BusSelector  OutputSignals=m,PIdq
  Bus Selector2 : BusSelector  OutputSignals=PrefPmeas,QrefQmeas
  Carriers Ap : Scope
  Demux : Demux  Outputs=2
  Demux1 : Demux  Outputs=2
  Gain : Gain  Gain=1e-6
  Gain1 : Gain  Gain=1e-6
  Gain2 : Gain  Gain=sqrt(3)/sqrt(2)*1e-3
  Gain3 : Gain  Gain=Pnom*1e-6
  Gain4 : Gain  Gain=Pnom*1e-6
  Iarm_A : Scope  NumInputPorts=2
  IdIq : Scope  NumInputPorts=2
  Ifilter_A : Scope
  Mux{1..5} (5 alike) : Mux  Inputs=2
  PQ_prim (MVA) : Scope  NumInputPorts=2
  PQmeas_MVA : Scope  NumInputPorts=2
  Power (Positive-Sequence) : spsPowerPositiveSequenceLib/Power (Positive-Sequence)  Freq=Fnom  Vinit=[0, 0]  Iinit=[0, 0]  Ts=Ts_Power
  Sequence Analyzer : spsSequenceAnalyzerLib/Sequence Analyzer  Freq=Fnom  n=1  seq=Positive  InInit=[1, 0]  Ts=Ts_Power
  Terminator{,1..14} (15 alike) : Terminator
  V12_ApAm : Scope  NumInputPorts=2
  V1_kVrmsLL_prim : Scope
  VIdc_Conv1 : Scope  NumInputPorts=2
  VIdc_Conv2 : Scope  NumInputPorts=2
  VIprim : Scope  NumInputPorts=2
  VIsec : Scope  NumInputPorts=2
  Vcap : Scope  NumInputPorts=2
  m  PIdq : Scope  NumInputPorts=2
  tag scope: P=global, Q=global, V1rmsLL=global
  wires:
  Mux5/1 -> Carriers Ap/1
  [Cr_Ap] -> Mux5/2
  [Uref_Ap] -> Mux5/1
  [Vc_Am] -> Vcap/2  "Am_mean"
  [Vc_Ap] -> Vcap/1  "Ap_mean"
  [Idc2] -> VIdc_Conv2/2  "I"
  [Vdc2] -> VIdc_Conv2/1  "V"
  Gain4/1 -> Demux1/1
  Gain3/1 -> Demux/1
  Mux2/1 -> PQmeas_MVA/2  "Qref Qmeas"
  Bus Selector2/2 -> Gain4/1  "<QrefQmeas>"
  Bus Selector2/1 -> Gain3/1  "<PrefPmeas>"
  Mux1/1 -> PQmeas_MVA/1  "Pref Pmeas"
  [meas1] -> Bus Selector2/1
  Gain2/1 -> V1_kVrmsLL_prim/1, [V1rmsLL]
  Gain1/1 -> PQ_prim (MVA)/2  "Mvar"
  Gain/1 -> PQ_prim (MVA)/1  "MW"
  [V12_Cm] -> Terminator14/1
  [V12_Bm] -> Terminator13/1
  [V12_Cp] -> Terminator12/1
  [V12_Bp] -> Terminator11/1
  [Ifilter_C] -> Terminator10/1
  [Ifilter_B] -> Terminator9/1
  Sequence Analyzer/1 -> Gain2/1
  Power (Positive-Sequence)/2 -> Gain1/1
  Power (Positive-Sequence)/1 -> Gain/1
  Sequence Analyzer/2 -> Terminator8/1
  [Iprim] -> Power (Positive-Sequence)/2
  [Vprim] -> Power (Positive-Sequence)/1, Sequence Analyzer/1
  [Idc1] -> VIdc_Conv1/2  "I"
  [Vdc1] -> VIdc_Conv1/1  "V"
  [Ifilter_A] -> Ifilter_A/1
  Bus Selector/4 -> Mux4/2  "<Iq>"
  Bus Selector/3 -> Mux4/1  "<Iqref>"
  Bus Selector/2 -> Mux3/2  "<Id>"
  Bus Selector/1 -> Mux3/1  "<Idref>"
  Mux4/1 -> IdIq/2  "Iqref  Iq"
  Mux3/1 -> IdIq/1  "Idref  Id"
  Bus Selector1/2 -> m  PIdq/2  "<PIdq>"
  Bus Selector1/1 -> m  PIdq/1  "<m>"
  [meas1] -> Bus Selector/1, Bus Selector1/1
  [I_Cm] -> Terminator7/1
  [I_Cp] -> Terminator6/1
  [I_Bm] -> Terminator5/1
  [I_Bp] -> Terminator4/1
  [I_Am] -> Iarm_A/2  "Am"
  [I_Ap] -> Iarm_A/1  "Ap"
  [Vc_Cm] -> Terminator3/1
  [Vc_Cp] -> Terminator2/1
  [Vc_Bm] -> Terminator1/1
  [Vc_Bp] -> Terminator/1
  [V12_Am] -> V12_ApAm/2  "Am"
  [V12_Ap] -> V12_ApAm/1  "Ap"
  [Vsec] -> VIsec/1  "V"
  [Isec] -> VIsec/2  "I"
  [Vprim] -> VIprim/1  "V"
  [Iprim] -> VIprim/2  "I"
  Demux/1 -> Mux1/1
  Demux/2 -> [P], Mux1/2
  Demux1/1 -> Mux2/1
  Demux1/2 -> [Q], Mux2/2

== system HVDCMMCInterconnection_O/Subsystem ==
  Current Measurement1 : spsCurrentMeasurementLib/Current Measurement  PhasorSimulation=off  OutputType=Complex  PSBequivalent=0
  Voltage Measurement : spsVoltageMeasurementLib/Voltage Measurement  PhasorSimulation=off  OutputType=Complex  PSBequivalent=0
  I1 : PMIOPort  Side=Left
  I2 : PMIOPort  Port=2  Side=Left
  O1 : PMIOPort  Port=3  Side=Right
  O2 : PMIOPort  Port=4  Side=Right
  tag scope: I_Ap=global, V12_Ap=global
  wires:
  Current Measurement1/1 -> [I_Ap]
  Voltage Measurement/1 -> [V12_Ap]
  connections:
  Current Measurement1/RConn1 -- Voltage Measurement/LConn1 -- I1/RConn1
  Current Measurement1/LConn1 -- O1/RConn1
  I2/RConn1 -- Voltage Measurement/LConn2 -- O2/RConn1

== system HVDCMMCInterconnection_O/Subsystem1 ==
  Current Measurement1 : spsCurrentMeasurementLib/Current Measurement  PhasorSimulation=off  OutputType=Complex  PSBequivalent=0
  Voltage Measurement : spsVoltageMeasurementLib/Voltage Measurement  PhasorSimulation=off  OutputType=Complex  PSBequivalent=0
  I1 : PMIOPort  Side=Left
  I2 : PMIOPort  Port=2  Side=Left
  O1 : PMIOPort  Port=3  Side=Right
  O2 : PMIOPort  Port=4  Side=Right
  tag scope: I_Am=global, V12_Am=global
  wires:
  Voltage Measurement/1 -> [V12_Am]
  Current Measurement1/1 -> [I_Am]
  connections:
  Voltage Measurement/LConn2 -- O2/RConn1 -- I2/RConn1
  Current Measurement1/LConn1 -- O1/RConn1
  Voltage Measurement/LConn1 -- Current Measurement1/RConn1 -- I1/RConn1

== system HVDCMMCInterconnection_O/Subsystem2 ==
  Current Measurement1 : spsCurrentMeasurementLib/Current Measurement  PhasorSimulation=off  OutputType=Complex  PSBequivalent=0
  Voltage Measurement : spsVoltageMeasurementLib/Voltage Measurement  PhasorSimulation=off  OutputType=Complex  PSBequivalent=0
  I1 : PMIOPort  Side=Left
  I2 : PMIOPort  Port=2  Side=Left
  O1 : PMIOPort  Port=3  Side=Right
  O2 : PMIOPort  Port=4  Side=Right
  tag scope: I_Bp=global, V12_Bp=global
  wires:
  Voltage Measurement/1 -> [V12_Bp]
  Current Measurement1/1 -> [I_Bp]
  connections:
  Voltage Measurement/LConn2 -- O2/RConn1 -- I2/RConn1
  Current Measurement1/LConn1 -- O1/RConn1
  Voltage Measurement/LConn1 -- Current Measurement1/RConn1 -- I1/RConn1

== system HVDCMMCInterconnection_O/Subsystem3 ==
  Current Measurement1 : spsCurrentMeasurementLib/Current Measurement  PhasorSimulation=off  OutputType=Complex  PSBequivalent=0
  Voltage Measurement : spsVoltageMeasurementLib/Voltage Measurement  PhasorSimulation=off  OutputType=Complex  PSBequivalent=0
  I1 : PMIOPort  Side=Left
  I2 : PMIOPort  Port=2  Side=Left
  O1 : PMIOPort  Port=3  Side=Right
  O2 : PMIOPort  Port=4  Side=Right
  tag scope: I_Bm=global, V12_Bm=global
  wires:
  Current Measurement1/1 -> [I_Bm]
  Voltage Measurement/1 -> [V12_Bm]
  connections:
  I1/RConn1 -- Current Measurement1/RConn1 -- Voltage Measurement/LConn1
  Current Measurement1/LConn1 -- O1/RConn1
  I2/RConn1 -- O2/RConn1 -- Voltage Measurement/LConn2

== system HVDCMMCInterconnection_O/Subsystem4 ==
  Current Measurement1 : spsCurrentMeasurementLib/Current Measurement  PhasorSimulation=off  OutputType=Complex  PSBequivalent=0
  Voltage Measurement : spsVoltageMeasurementLib/Voltage Measurement  PhasorSimulation=off  OutputType=Complex  PSBequivalent=0
  I1 : PMIOPort  Side=Left
  I2 : PMIOPort  Port=2  Side=Left
  O1 : PMIOPort  Port=3  Side=Right
  O2 : PMIOPort  Port=4  Side=Right
  tag scope: I_Cp=global, V12_Cp=global
  wires:
  Current Measurement1/1 -> [I_Cp]
  Voltage Measurement/1 -> [V12_Cp]
  connections:
  I1/RConn1 -- Current Measurement1/RConn1 -- Voltage Measurement/LConn1
  Current Measurement1/LConn1 -- O1/RConn1
  I2/RConn1 -- O2/RConn1 -- Voltage Measurement/LConn2

== system HVDCMMCInterconnection_O/Subsystem5 ==
  Current Measurement1 : spsCurrentMeasurementLib/Current Measurement  PhasorSimulation=off  OutputType=Complex  PSBequivalent=0
  Voltage Measurement : spsVoltageMeasurementLib/Voltage Measurement  PhasorSimulation=off  OutputType=Complex  PSBequivalent=0
  I1 : PMIOPort  Side=Left
  I2 : PMIOPort  Port=2  Side=Left
  O1 : PMIOPort  Port=3  Side=Right
  O2 : PMIOPort  Port=4  Side=Right
  tag scope: I_Cm=global, V12_Cm=global
  wires:
  Voltage Measurement/1 -> [V12_Cm]
  Current Measurement1/1 -> [I_Cm]
  connections:
  Voltage Measurement/LConn2 -- O2/RConn1 -- I2/RConn1
  Current Measurement1/LConn1 -- O1/RConn1
  Voltage Measurement/LConn1 -- Current Measurement1/RConn1 -- I1/RConn1

== system HVDCMMCInterconnection_O/param ==

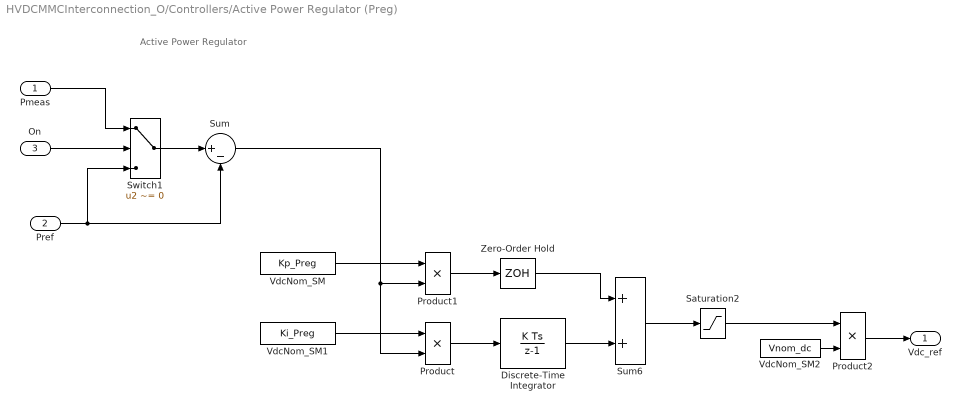
== system HVDCMMCInterconnection_O/Controllers/Active Power Regulator (Preg) ==
  note: Active Power Regulator
  Pmeas : Inport  PortDimensions=1
  Pref : Inport  Port=2  PortDimensions=1  SampleTime=Ts
  On : Inport  Port=3  PortDimensions=1  SampleTime=Ts
  Discrete-Time Integrator : DiscreteIntegrator  InitialCondition=1  SampleTime=Ts  LimitOutput=on  UpperSaturationLimit=Limits_Preg(1)  LowerSaturationLimit=Limits_Preg(2)  ICPrevOutput=DiscIntNeverNeededParam  ICPrevScaledInput=DiscIntNeverNeededParam
  Product : Product  RndMeth=Zero
  Product1 : Product  RndMeth=Zero
  Product2 : Product
  Saturation2 : Saturate  UpperLimit=Limits_Preg(1)  LowerLimit=Limits_Preg(2)  SampleTime=Ts
  Sum : Sum  Inputs=|+-
  Sum6 : Sum  InputSameDT=on  SaturateOnIntegerOverflow=on  SampleTime=Ts  OutDataTypeStr=Inherit: Same as first input
  Switch1 : Switch  Criteria=u2 ~= 0  Threshold=0.5  OutDataTypeStr=double  SaturateOnIntegerOverflow=off  InputSameDT=off
  VdcNom_SM : Constant  Value=Kp_Preg  SampleTime=Ts
  VdcNom_SM1 : Constant  Value=Ki_Preg  SampleTime=Ts
  VdcNom_SM2 : Constant  Value=Vnom_dc  SampleTime=Ts
  Zero-Order Hold : ZeroOrderHold  SampleTime=Ts
  Vdc_ref : Outport  SampleTime=Ts
  wires:
  Product2/1 -> Vdc_ref/1
  VdcNom_SM2/1 -> Product2/2
  Pmeas/1 -> Switch1/1
  On/1 -> Switch1/2
  Switch1/1 -> Sum/1
  Pref/1 -> Switch1/3, Sum/2
  Zero-Order Hold/1 -> Sum6/1
  Discrete-Time Integrator/1 -> Sum6/2
  Sum6/1 -> Saturation2/1
  VdcNom_SM1/1 -> Product/1
  Product1/1 -> Zero-Order Hold/1
  Product/1 -> Discrete-Time Integrator/1
  VdcNom_SM/1 -> Product1/1
  Saturation2/1 -> Product2/1
  Sum/1 -> Product1/2, Product/2

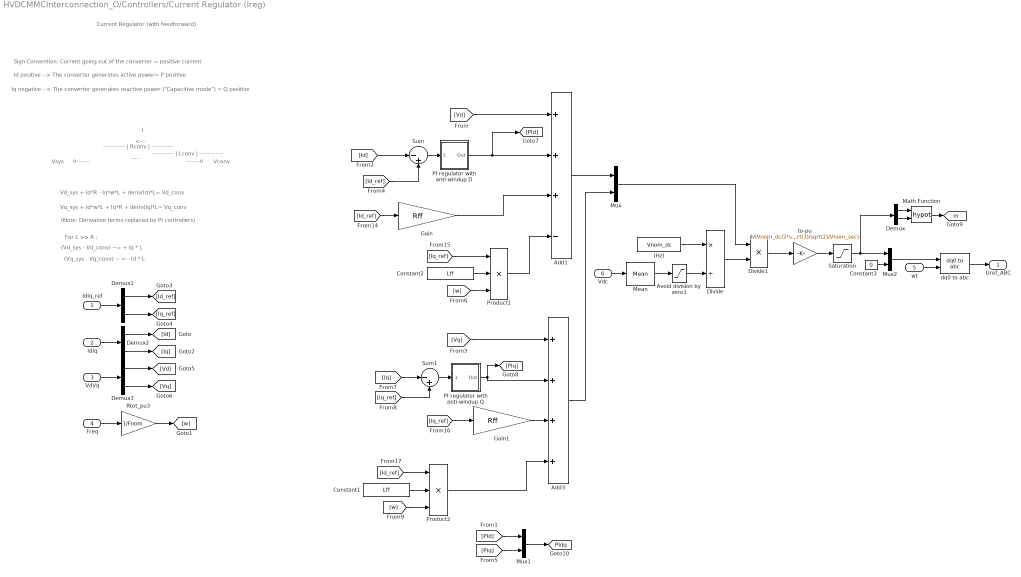
== system HVDCMMCInterconnection_O/Controllers/Current Regulator (Ireg) ==
  note: -----------
      | | Lconv |
      | ------------
  note: <---
  note: -------o
  note: Vconv
  note: ----
  note: -----------
      | | Rconv |
      | -----------
  note: For L >> R :
  note: (Vq_sys - Vq_conv) ~ = - Id * L
  note: (Vd_sys - Vd_conv) ~= + Iq * L
  note: Id positive --> The converter generates active power= P positive
  note: Iq negative --> The converter generates reactive power ("Capacitive mode") = Q positive
  note: Sign Convention: Current going out of the converter = positive current
  note: Current Regulator
      | (with feedforward)
  note: Vq_sys + Id*w*L + Iq*R + deriv(Iq)*L= Vq_conv
  note: Vd_sys + Id*R - Iq*w*L + deriv(Id)*L= Vd_conv
  note: (Note: Derivative terms replaced by PI controllers)
  note: Vsys
  note: o-------
  note: I
  IdIq_ref : Inport  PortDimensions=2
  IdIq : Inport  Port=2  PortDimensions=2
  VdVq : Inport  Port=3  PortDimensions=2
  Freq : Inport  Port=4  PortDimensions=1
  wt : Inport  Port=5  PortDimensions=1
  Vdc : Inport  Port=6  PortDimensions=1
  " (Hz)" : Constant  Value=Vnom_dc  SampleTime=Ts
  Add1 : Sum  Inputs=+++-
  Add3 : Sum  Inputs=++++
  Avoid division by zero1 : Saturate  UpperLimit=Vnom_dc*1.25  LowerLimit=Vnom_dc*0.75
  Constant1 : Constant  Value=Lff  SampleTime=Ts_Control
  Constant2 : Constant  Value=Lff  SampleTime=Ts_Control
  Constant3 : Constant  Value=0  SampleTime=Ts
  Demux{,1..3} (4 alike) : Demux  Outputs=2
  Divide : Product  Inputs=*/
  Divide1 : Product  Inputs=**
  Gain : Gain  Gain=Rff
  Gain1 : Gain  Gain=Rff
  Math Function : Math  Operator=hypot  SignedPower=on
  Mean : spsMeanLib/Mean  Freq=Fnom/3  Vinit=Vnom_dc  Ts=Ts
  Mux : Mux  Inputs=2
  Mux1 : Mux  Inputs=2
  Mux2 : Mux  Inputs=[2 1]
  PI regulator with anti-windup D : Subsystem  DialogController=POWERSYS.PowerSysDialog  mask(Discrete PI Controller){Kp=Kp_Ireg, Ki=Ki_Ireg, Par_Limits=Limits_Ireg, Init=0, Ts=Ts}
      mask prompts: Kp "Proportional gain (Kp):"; Ki "Integral gain (Ki):"; Par_Limits "Output limits: [ Upper   Lower ]"; Init "Output initial value:"; Ts "Sample time:"
      mask help: This block implements a discrete PI controller.
      mask init:
      | UpperLimit=Par_Limits(1);
      | LowerLimit=Par_Limits(2);
      | power_initmask();
      mask Help: This block is part of a subset of blocks in the Extras library that does not have documentation associated with it, other than the block mask description.
      mask Display: disp('PI');
  PI regulator with anti-windup Q : Subsystem  DialogController=POWERSYS.PowerSysDialog  mask(Discrete PI Controller){Kp=Kp_Ireg, Ki=Ki_Ireg, Par_Limits=Limits_Ireg, Init=0, Ts=Ts}
      mask prompts: Kp "Proportional gain (Kp):"; Ki "Integral gain (Ki):"; Par_Limits "Output limits: [ Upper   Lower ]"; Init "Output initial value:"; Ts "Sample time:"
      mask help: This block implements a discrete PI controller.
      mask init:
      | UpperLimit=Par_Limits(1);
      | LowerLimit=Par_Limits(2);
      | power_initmask();
      mask Help: This block is part of a subset of blocks in the Extras library that does not have documentation associated with it, other than the block mask description.
      mask Display: disp('PI');
  Product1 : Product  Inputs=3  RndMeth=Zero
  Product2 : Product  Inputs=3  RndMeth=Zero
  Rtot_pu3 : Gain  Gain=1/Fnom  SaturateOnIntegerOverflow=on  OutDataTypeStr=Inherit: Same as input  ParamDataTypeStr=Inherit: Same as input
  Saturation : Saturate  UpperLimit=Limits_Ireg(1)  LowerLimit=Limits_Ireg(2)
  Sum : Sum  Inputs=|-+
  Sum1 : Sum  Inputs=|-+
  dq0 to abc : spsdq0toabcLib/dq0 to abc  Alignment=90 degrees behind phase A axis
  to-pu : Gain  Gain=1/(Vnom_dc/2*sqrt(3)/sqrt(2)/Vnom_sec)
  Uref_ABC : Outport
  tag scope: PIdq=global, m=global
  wires:
  wt/1 -> dq0 to abc/2
  to-pu/1 -> Saturation/1
  Mux/1 -> Divide1/1
  dq0 to abc/1 -> Uref_ABC/1
  Divide/1 -> Divide1/2
  Mean/1 -> Avoid division by zero1/1
  Divide1/1 -> to-pu/1
  " (Hz)"/1 -> Divide/1
  Vdc/1 -> Mean/1
  Avoid division by zero1/1 -> Divide/2
  Mux1/1 -> [PIdq]
  Constant3/1 -> Mux2/2
  Mux2/1 -> dq0 to abc/1
  Demux/2 -> Math Function/2
  Demux/1 -> Math Function/1
  Math Function/1 -> [m]
  Saturation/1 -> Mux2/1, Demux/1
  PI regulator with anti-windup D/1(Out) -> [PId], Add1/2
  PI regulator with anti-windup Q/1(Out) -> [PIq], Add3/2
  [Vd] -> Add1/1
  Product1/1 -> Add1/4
  Gain/1 -> Add1/3
  Gain1/1 -> Add3/3
  Product2/1 -> Add3/4
  [Vq] -> Add3/1
  Demux2/1 -> [Id]
  IdIq/1 -> Demux2/1
  [Id_ref] -> Product2/1
  [Iq_ref] -> Gain1/1
  [Iq_ref] -> Product1/1
  [Id_ref] -> Gain/1
  [Id] -> Sum/1
  [Iq] -> Sum1/1
  Demux2/2 -> [Iq]
  [PIq] -> Mux1/2
  [PId] -> Mux1/1
  [w] -> Product1/3
  Constant2/1 -> Product1/2
  [w] -> Product2/3
  Constant1/1 -> Product2/2
  [Iq_ref] -> Sum1/2
  Sum1/1 -> PI regulator with anti-windup Q/1(Error)
  [Id_ref] -> Sum/2
  Sum/1 -> PI regulator with anti-windup D/1(Error)
  VdVq/1 -> Demux3/1
  Demux3/2 -> [Vq]
  Demux3/1 -> [Vd]
  IdIq_ref/1 -> Demux1/1
  Demux1/2 -> [Iq_ref]
  Demux1/1 -> [Id_ref]
  Rtot_pu3/1 -> [w]
  Freq/1 -> Rtot_pu3/1
  Add1/1 -> Mux/1
  Add3/1 -> Mux/2

== system HVDCMMCInterconnection_O/Controllers/DC Voltage Regulator (VDCreg) ==
  note: VDC Regulator
  Vdc_meas : Inport  PortDimensions=1
  Vdc_ref : Inport  Port=2  PortDimensions=1
  On : Inport  Port=3  PortDimensions=1
  Discrete-Time Integrator : DiscreteIntegrator  SampleTime=Ts  LimitOutput=on  UpperSaturationLimit=Limits_VDCreg(1)  LowerSaturationLimit=Limits_VDCreg(2)  ICPrevOutput=DiscIntNeverNeededParam  ICPrevScaledInput=DiscIntNeverNeededParam
  Product : Product  RndMeth=Zero
  Product1 : Product  RndMeth=Zero
  Rtot_pu2 : Gain  Gain=1/Vnom_dc  SaturateOnIntegerOverflow=on  OutDataTypeStr=Inherit: Same as input  ParamDataTypeStr=Inherit: Same as input
  Saturation2 : Saturate  UpperLimit=Limits_VDCreg(1)  LowerLimit=Limits_VDCreg(2)  SampleTime=Ts
  Sum : Sum  Inputs=|+-
  Sum6 : Sum  InputSameDT=on  SaturateOnIntegerOverflow=on  SampleTime=Ts  OutDataTypeStr=Inherit: Same as first input
  Switch1 : Switch  Criteria=u2 ~= 0  Threshold=0.5  OutDataTypeStr=double  SaturateOnIntegerOverflow=off  InputSameDT=off
  VdcNom_SM : Constant  Value=Kp_VDCreg
  VdcNom_SM1 : Constant  Value=Ki_VDCreg
  Zero-Order Hold : ZeroOrderHold  SampleTime=Ts
  Id_ref : Outport
  wires:
  Rtot_pu2/1 -> Product/2, Product1/2
  Saturation2/1 -> Id_ref/1
  VdcNom_SM/1 -> Product1/1
  Product/1 -> Discrete-Time Integrator/1
  Product1/1 -> Zero-Order Hold/1
  VdcNom_SM1/1 -> Product/1
  Sum6/1 -> Saturation2/1
  Discrete-Time Integrator/1 -> Sum6/2
  Zero-Order Hold/1 -> Sum6/1
  Vdc_ref/1 -> Sum/2, Switch1/3
  Switch1/1 -> Sum/1
  On/1 -> Switch1/2
  Sum/1 -> Rtot_pu2/1
  Vdc_meas/1 -> Switch1/1
